simulink model "sprawko3simulink"  (R2020b)
settings: Solver=VariableStepAuto  StartTime=0.0  StopTime=10.0  RelTol=1e-3
values from neighbouring files (symbols this model uses):
  cv1 = ro*cp*v1    (= 108540)    [zaj1.m]
  cv2 = ro*cp*v2    (= 36180)    [zaj1.m]
  dqg = 1000    [zaj1.m]
  dT2N = 5    [zaj1.m]
  dTzew = 0    [zaj1.m]
  k = 1.75/dqg    (= 0.00175)    [zaj1.m]
  Kp_chien0 = (0.35*T)/(k*T_0)*4.49    (= 26940)    [zaj1.m]
  Kp_chien20 = (0.6*T)/(k*T_0)    (= 10285.7142857)    [zaj1.m]
  Kp_nichols = (0.9*T)/(k*T_0)    (= 15428.5714286)    [zaj1.m]
  Ks0 = (Ks2*(T2N-TzewN))/(T1N-T2N)    (= 903.225806452)    [zaj1.m]
  Ks1 = 3*Ks2    (= 387.096774194)    [zaj1.m]
  Ks2 = QgN/(3*(T1N-TzewN)+T2N-TzewN)    (= 129.032258065)    [zaj1.m]
  QgN = 20000    [zaj1.m]
  steptime = 100    [zaj1.m]
  T = 300    [zaj1.m]
  T1N = 20    [zaj1.m]
  T2N = 15    [zaj1.m]
  T_0 = 10    [zaj1.m]
  Ti_chien0 = 1.2*T    (= 360)    [zaj1.m]
  Ti_chien20 = T    (= 300)    [zaj1.m]
  Ti_nichols = 3.33*T_0    (= 33.3)    [zaj1.m]
  tw10d = [cv1*cv2 cv1*Ks0+cv1*Ks2+Ks1*cv2+Ks0*cv2 Ks0*Ks1+Ks2*Ks0+Ks1*Ks2]    [zaj1.m]
  tw1intinit = T1N    (= 20)    [zaj1.m]
  tw2intinit = T2N    (= 15)    [zaj1.m]
  TzewN = -20    [zaj1.m]
settings Model: Creator=bilin  LastModifiedBy=bilin

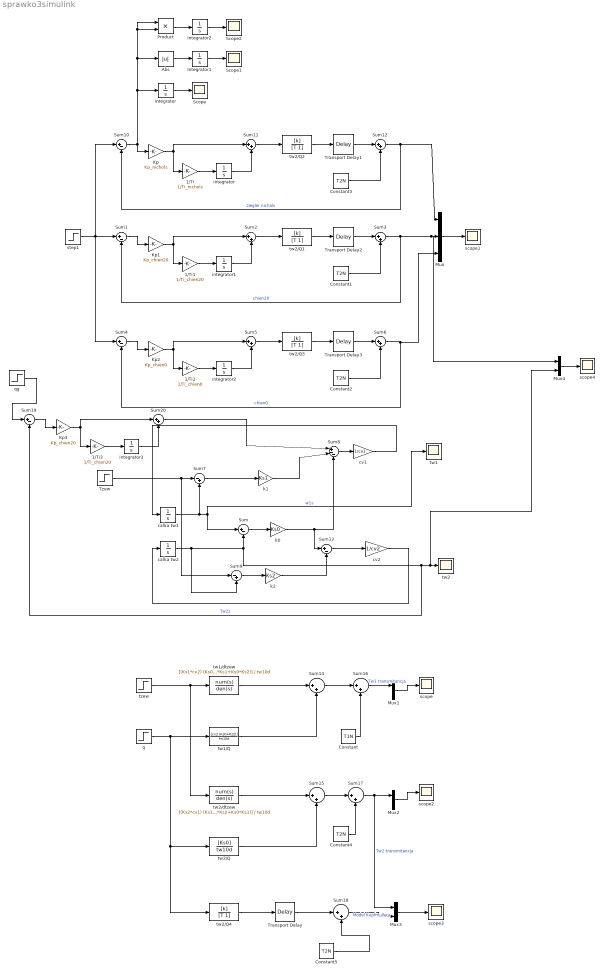
== system sprawko3simulink ==
  1/Ti : Gain  Gain=1/Ti_nichols
  1/Ti1 : Gain  Gain=1/Ti_chien20
  1/Ti2 : Gain  Gain=1/Ti_chien0
  1/Ti3 : Gain  Gain=1/Ti_chien20
  Abs : Abs
  Constant : Constant  Value=T1N
  Constant{1..5} (5 alike) : Constant  Value=T2N
  Integrator : Integrator
  Integrator1 : Integrator
  Integrator2 : Integrator
  Kp : Gain  Gain=Kp_nichols
  Kp1 : Gain  Gain=Kp_chien20
  Kp2 : Gain  Gain=Kp_chien0
  Kp3 : Gain  Gain=Kp_chien20
  Mux : Mux  Inputs=3
  Mux{1..4} (4 alike) : Mux  Inputs=2
  Product : Product
  Scope : Scope
  Scope1 : Scope
  Scope2 : Scope
  Sum{,1,4,10,13,19} (6 alike) : Sum  Inputs=|+-
  Sum{2..3,5..6,11..12,14..18,20} (12 alike) : Sum  Inputs=|++
  Sum7 : Sum  Inputs=|-+
  Sum8 : Sum  Inputs=|+--
  Sum9 : Sum  Inputs=|-+
  Transport Delay{,1..3} (4 alike) : TransportDelay  DelayTime=T_0
  Tzew : Step  Time=100  Before=TzewN  After=TzewN+dTzew  SampleTime=0
  calka tw1 : Integrator  InitialCondition=tw1intinit
  calka tw2 : Integrator  InitialCondition=tw2intinit
  cv1 : Gain  Gain=1/cv1
  cv2 : Gain  Gain=1/cv2
  integrator : Integrator
  integrator1 : Integrator
  integrator2 : Integrator
  integrator3 : Integrator  InitialCondition=QgN
  k0 : Gain  Gain=Ks0
  k1 : Gain  Gain=Ks1
  k2 : Gain  Gain=Ks2
  q : Step  Time=steptime  After=dqg  SampleTime=0
  qg : Step  Time=100  Before=T2N  After=T2N+dT2N  SampleTime=0
  scope{,1..4} (5 alike) : Scope
  step1 : Step  Time=100  Before=T2N  After=T2N+dT2N  SampleTime=0
  tw1 : Scope
  tw1/Q : TransferFcn  Numerator=[cv2 (Ks0+Ks2)]  Denominator=tw10d
  tw1/dtzew : TransferFcn  Numerator=[(Ks1*cv2) (Ks0*Ks1+Ks2*Ks1+Ks0*Ks2)]  Denominator=tw10d
  tw2 : Scope
  tw2/Q : TransferFcn  Numerator=[Ks0]  Denominator=tw10d
  tw2/Q{1..4} (4 alike) : TransferFcn  Numerator=[k]  Denominator=[T 1]
  tw2/dtzew : TransferFcn  Numerator=[(Ks2*cv1) (Ks1*Ks2+Ks0*Ks2+Ks0*Ks1)]  Denominator=tw10d
  tzew : Step  Time=steptime  After=dTzew  SampleTime=0
  wires:
  k0/1 -> Sum13/1, Sum8/3
  Constant3/1 -> Sum12/2
  Transport Delay3/1 -> Sum6/1
  Sum15/1 -> Sum17/1
  k2/1 -> Sum13/2
  Kp3/1 -> Sum20/1, 1/Ti3/1
  Mux1/1 -> scope/1
  calka tw1/1 -> Sum7/2, tw1/1, Sum/1  "w1s"
  1/Ti2/1 -> integrator2/1
  Sum/1 -> k0/1
  integrator1/1 -> Sum2/2
  tw2/Q1/1 -> Transport Delay2/1
  integrator3/1 -> Sum20/2
  cv2/1 -> calka tw2/1
  Sum8/1 -> cv1/1
  Sum3/1 -> Sum1/2, Mux4/1, Mux/2  "chien20"
  Sum7/1 -> k1/1
  tw2/Q/1 -> Sum15/2
  Mux2/1 -> scope2/1
  Sum1/1 -> Kp1/1
  Mux/1 -> scope1/1
  Sum18/1 -> Mux3/2  "Model Kupfmullera"
  Sum14/1 -> Sum16/1
  Sum13/1 -> cv2/1
  tw2/dtzew/1 -> Sum15/1
  Integrator2/1 -> Scope2/1
  tw1/dtzew/1 -> Sum14/1
  tw1/Q/1 -> Sum14/2
  Sum17/1 -> Mux2/1, Mux3/1  "Tw2 transmitancja"
  Mux3/1 -> scope3/1
  Transport Delay/1 -> Sum18/1
  Kp/1 -> Sum11/1, 1/Ti/1
  Constant5/1 -> Sum18/2
  Transport Delay2/1 -> Sum3/1
  Constant4/1 -> Sum17/2
  Constant/1 -> Sum16/2
  Kp1/1 -> Sum2/1, 1/Ti1/1
  Product/1 -> Integrator2/1
  integrator2/1 -> Sum5/2
  Integrator/1 -> Scope/1
  Kp2/1 -> Sum5/1, 1/Ti2/1
  Integrator1/1 -> Scope1/1
  tw2/Q2/1 -> Transport Delay1/1
  tzew/1 -> tw2/dtzew/1, tw1/dtzew/1
  Sum2/1 -> tw2/Q1/1
  Constant1/1 -> Sum3/2
  1/Ti/1 -> integrator/1
  Sum11/1 -> tw2/Q2/1
  Tzew/1 -> Sum9/1, Sum7/1
  Sum10/1 -> Product/1, Product/2, Abs/1, Integrator/1, Kp/1
  q/1 -> tw2/Q/1, tw2/Q4/1, tw1/Q/1
  Abs/1 -> Integrator1/1
  Sum12/1 -> Sum10/2, Mux/1  "ziegler nichols"
  Sum4/1 -> Kp2/1
  Sum19/1 -> Kp3/1
  cv1/1 -> calka tw1/1
  Sum5/1 -> tw2/Q3/1
  Sum9/1 -> k2/1
  k1/1 -> Sum8/2
  tw2/Q4/1 -> Transport Delay/1
  tw2/Q3/1 -> Transport Delay3/1
  Mux4/1 -> scope4/1
  1/Ti3/1 -> integrator3/1
  calka tw2/1 -> Sum9/2, Mux4/2, tw2/1, Sum19/2, Sum/2  "Tw2s"
  Sum6/1 -> Mux/3, Sum4/2  "chien0"
  integrator/1 -> Sum11/2
  Sum20/1 -> Sum8/1
  Sum16/1 -> Mux1/1  "Tw1 transmitancja"
  1/Ti1/1 -> integrator1/1
  Constant2/1 -> Sum6/2
  Transport Delay1/1 -> Sum12/1
  step1/1 -> Sum10/1, Sum4/1, Sum1/1
  qg/1 -> Sum19/1
